simulink model "axemplul1"  (Simulink 7.2)
settings: Solver=ode45  StartTime=0.0  StopTime=10.0  RelTol=1e-3
settings Model: Creator=Student  LastModifiedBy=Student

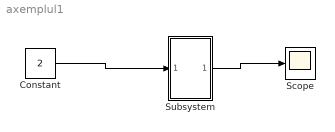
== system axemplul1 ==
  Constant : Constant  Value=2  OutDataType=sfix(16)  OutScaling=2^0
  Scope : Scope
  Subsystem : Subsystem  mask{m=3, b=2}
      mask prompts: m "panta"; b "constanta"
  wires:
  Constant/1 -> Subsystem/1(In1)
  Subsystem/1(Out1) -> Scope/1

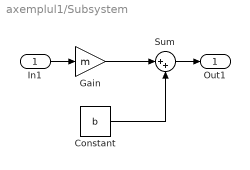
== system axemplul1/Subsystem ==
  In1 : Inport
  Constant : Constant  Value=b  OutDataType=sfix(16)  OutScaling=2^0
  Gain : Gain  Gain=m  ParameterDataType=sfix(16)  ParameterScaling=2^0  OutDataType=sfix(16)  OutScaling=2^0
  Sum : Sum  Inputs=|++  OutDataType=sfix(16)  OutScaling=2^0
  Out1 : Outport
  wires:
  Gain/1 -> Sum/1
  Constant/1 -> Sum/2
  In1/1 -> Gain/1
  Sum/1 -> Out1/1
